simulink model "Flex_Satellite"  (R2018b)
settings: Solver=VariableStepAuto  StartTime=0.0  StopTime=10.0  RelTol=1e-3
values from neighbouring files (symbols this model uses):
  alpha = 0.5736    [constants.m]
  c_damp = 0.00495    [constants.m]
  J_s = 31.38    [constants.m]
  w_mode = 2.6268    [constants.m]
settings Model: Creator=Yavuz  LastModifiedBy=ohara
settings DebuggingCC: AlgebraicLoopMsg=none

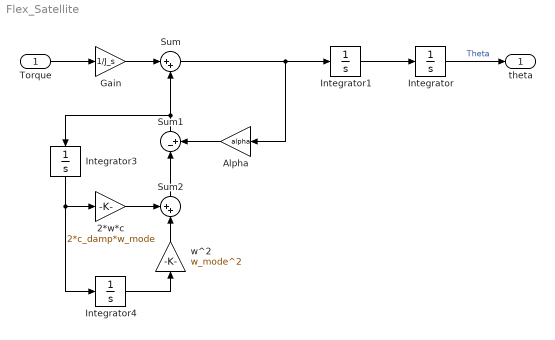
== system Flex_Satellite ==
  Torque : Inport
  2*w*c : Gain  Gain=2*c_damp*w_mode
  Alpha : Gain  Gain=alpha
  Gain : Gain  Gain=1/J_s
  Integrator{,1,3..4} (4 alike) : Integrator
  Sum : Sum  Inputs=|++
  Sum1 : Sum  Inputs=|-+
  Sum2 : Sum  Inputs=++|
  w^2 : Gain  Gain=w_mode^2
  theta : Outport
  wires:
  Integrator/1 -> theta/1  "Theta"
  Integrator1/1 -> Integrator/1
  Torque/1 -> Gain/1
  Gain/1 -> Sum/1
  Sum/1 -> Integrator1/1, Alpha/1
  Sum1/1 -> Integrator3/1, Sum/2
  Alpha/1 -> Sum1/2
  Sum2/1 -> Sum1/1
  2*w*c/1 -> Sum2/1
  Integrator3/1 -> Integrator4/1, 2*w*c/1
  w^2/1 -> Sum2/2
  Integrator4/1 -> w^2/1
